simulink model "model"  (R2020b)
settings: Solver=VariableStepAuto  StartTime=0.0  StopTime=10.0  RelTol=1e-3
settings Model: Creator=Lenovo  LastModifiedBy=Lenovo

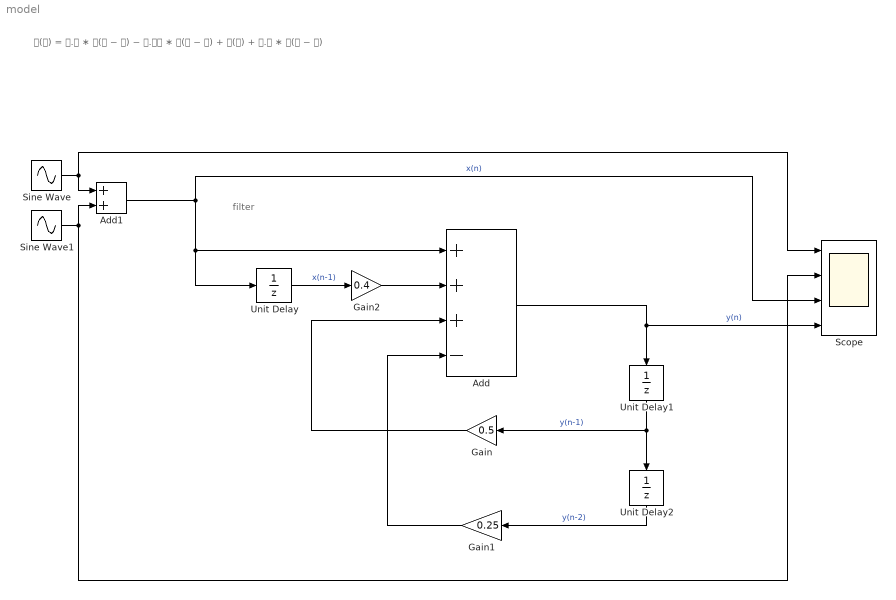
== system model ==
  note: filter
  note: 𝐲(𝐧) = 𝟎.𝟓 ∗ 𝐲(𝐧 − 𝟏) − 𝟎.𝟐𝟓 ∗ 𝐲(𝐧 − 𝟐) + 𝐱(𝐧) + 𝟎.𝟒 ∗ 𝐱(𝐧 − 𝟏)
  Add : Sum  Inputs=+++-
  Add1 : Sum
  Gain : Gain  Gain=0.5
  Gain1 : Gain  Gain=0.25
  Gain2 : Gain  Gain=0.4
  Scope : Scope  NumInputPorts=4
  Sine Wave : Sin  SampleTime=0
  Sine Wave1 : Sin  Amplitude=0.5  Frequency=50  SampleTime=0
  Unit Delay : UnitDelay  SampleTime=-1  HasFrameUpgradeWarning=on
  Unit Delay1 : UnitDelay  SampleTime=-1  HasFrameUpgradeWarning=on
  Unit Delay2 : UnitDelay  SampleTime=-1  HasFrameUpgradeWarning=on
  wires:
  Add1/1 -> Add/1, Unit Delay/1, Scope/3  "x(n)"
  Unit Delay2/1 -> Gain1/1  "y(n-2)"
  Unit Delay/1 -> Gain2/1  "x(n-1)"
  Gain/1 -> Add/3
  Gain1/1 -> Add/4
  Gain2/1 -> Add/2
  Add/1 -> Scope/4, Unit Delay1/1  "y(n)"
  Unit Delay1/1 -> Gain/1, Unit Delay2/1  "y(n-1)"
  Sine Wave/1 -> Scope/1, Add1/1
  Sine Wave1/1 -> Scope/2, Add1/2
